simulink model "ABS_003"  (R2020b)
settings: Solver=VariableStepAuto  StartTime=0.0  StopTime=20  RelTol=1e-3
model workspace: external: MAT-File component_values.mat (data not in the file)
values from neighbouring files (symbols this model uses):
  g = 9.81    [component_values.mat]
  I = 5    [component_values.mat]
  m = 75    [component_values.mat]
  R = 1.25    [component_values.mat]
  Rr = 1.25    [component_values.mat]
  v0 = 44    [component_values.mat]
libraries: pid_lib x1
settings Model: Creator=Liu  LastModifiedBy=Quincy.liu
settings OptimizationCC: LifeSpan=inf
settings DebuggingCC: ArithmeticOperatorsInVariantConditions=warning
settings SFSimCC: CustomCodeUndefinedFunction=UseInterfaceOnly
settings CodeAppCC: StateflowObjectComments=on

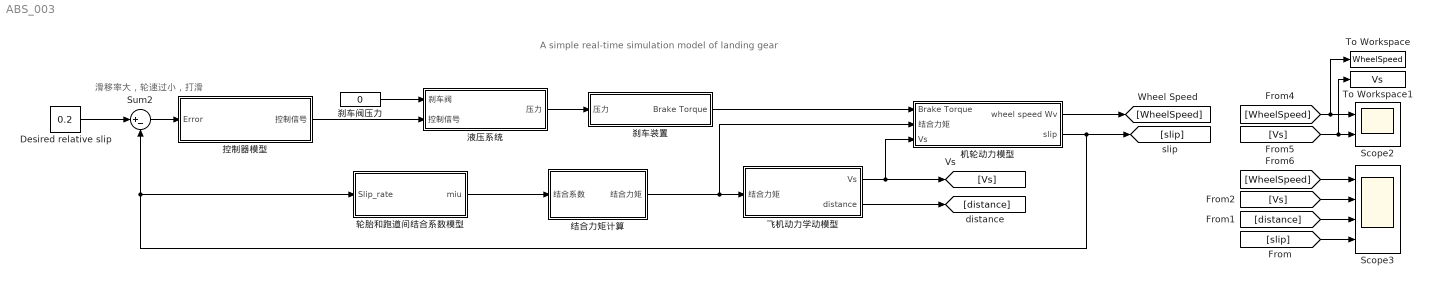
== system ABS_003 ==
  note: A simple real-time simulation model of landing gear
  note: 滑移率大，轮速过小，打滑
  Desired relative slip : Constant  Value=0.2
  Scope2 : Scope  NumInputPorts=2
  Scope3 : Scope  NumInputPorts=4
  Sum2 : Sum  Inputs=|+-  InputSameDT=on  SaturateOnIntegerOverflow=on  OutDataTypeStr=Inherit: Same as first input
  To Workspace : ToWorkspace  VariableName=WheelSpeed  SampleTime=-1
  To Workspace1 : ToWorkspace  VariableName=Vs  SaveFormat=Timeseries  SampleTime=-1
  刹车装置 : Subsystem
  刹车阀压力 : Constant  Value=0
  控制器模型 : Subsystem  Variant=on  VariantControlMode=label  LabelModeActiveChoice=Variant1
  "机轮动力模型 " : Subsystem
  液压系统 : Subsystem
  结合力矩计算 : Subsystem
  轮胎和跑道间结合系数模型 : Subsystem
  飞机动力学动模型 : Subsystem
  wires:
  Desired relative slip/1 -> Sum2/1
  结合力矩计算/1(结合力矩) -> 飞机动力学动模型/1(结合力矩), "机轮动力模型 "/2(结合力矩)
  轮胎和跑道间结合系数模型/1(miu) -> 结合力矩计算/1(结合系数)
  飞机动力学动模型/1(Vs) -> [Vs], "机轮动力模型 "/3(Vs)
  飞机动力学动模型/2(distance) -> [distance]
  Sum2/1 -> 控制器模型/1(Error)
  控制器模型/1(控制信号) -> 液压系统/2(控制信号)
  液压系统/1(压力) -> 刹车装置/1(压力)
  刹车装置/1(Brake Torque) -> "机轮动力模型 "/1(Brake Torque)
  "机轮动力模型 "/2(slip) -> [slip], 轮胎和跑道间结合系数模型/1(Slip_rate), Sum2/2
  [slip] -> Scope3/4
  [distance] -> Scope3/3
  [Vs] -> Scope3/2
  "机轮动力模型 "/1(wheel speed Wv) -> [WheelSpeed]
  [Vs] -> To Workspace1/1, Scope2/2
  [WheelSpeed] -> To Workspace/1, Scope2/1
  [WheelSpeed] -> Scope3/1
  刹车阀压力/1 -> 液压系统/1(刹车阀)

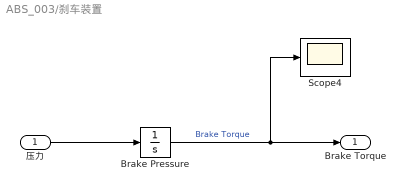
== system ABS_003/刹车装置 ==
  压力 : Inport
  Brake Pressure : Integrator  LimitOutput=on  UpperSaturationLimit=1000  LowerSaturationLimit=0
  Scope4 : Scope
  Brake Torque : Outport
  wires:
  Brake Pressure/1 -> Brake Torque/1, Scope4/1  "Brake Torque"
  压力/1 -> Brake Pressure/1

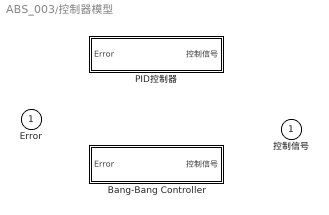
== system ABS_003/控制器模型 ==
  Error : Inport
  "Bang-Bang Controller " : Subsystem  VariantControl=Variant2
  PID控制器 : Subsystem  TreatAsAtomicUnit=on  VariantControl=Variant1
  控制信号 : Outport

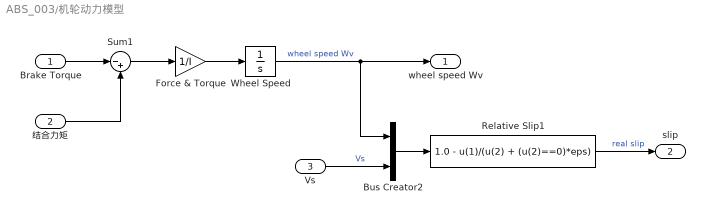
== system ABS_003/机轮动力模型  ==
  Brake Torque : Inport
  结合力矩 : Inport  Port=2
  Vs : Inport  Port=3
  Bus Creator2 : BusCreator  Inputs=2
  Force & Torque : Gain  Gain=1/I
  Relative Slip1 : Fcn  Expr=1.0 - u(1)/(u(2) + (u(2)==0)*eps)
  Sum1 : Sum  Inputs=|-+
  Wheel Speed : Integrator  InitialCondition=v0/R  LimitOutput=on  UpperSaturationLimit=1000  LowerSaturationLimit=0
  wheel speed Wv : Outport
  slip : Outport  Port=2
  wires:
  Force & Torque/1 -> Wheel Speed/1
  结合力矩/1 -> Sum1/2
  Sum1/1 -> Force & Torque/1
  Brake Torque/1 -> Sum1/1
  Vs/1 -> Bus Creator2/2  "Vs"
  Bus Creator2/1 -> Relative Slip1/1
  Relative Slip1/1 -> slip/1  "real slip"
  Wheel Speed/1 -> Bus Creator2/1, wheel speed Wv/1  "wheel speed Wv"

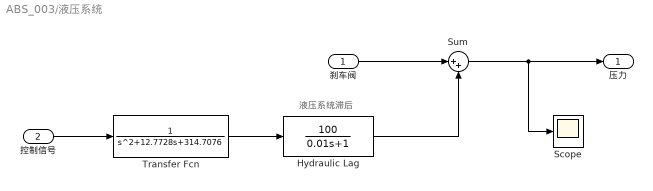
== system ABS_003/液压系统 ==
  note: 液压系统滞后
  刹车阀 : Inport
  控制信号 : Inport  Port=2
  Hydraulic Lag : TransferFcn  Numerator=[100]  Denominator=[0.01 1]
  Scope : Scope
  Sum : Sum  Inputs=|++
  Transfer Fcn : TransferFcn  Denominator=[1 12.7728 314.7076]
  压力 : Outport
  wires:
  控制信号/1 -> Transfer Fcn/1
  Transfer Fcn/1 -> Hydraulic Lag/1
  Hydraulic Lag/1 -> Sum/2
  刹车阀/1 -> Sum/1
  Sum/1 -> Scope/1, 压力/1

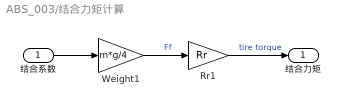
== system ABS_003/结合力矩计算 ==
  结合系数 : Inport
  Rr1 : Gain  Gain=Rr  SaturateOnIntegerOverflow=on  OutDataTypeStr=Inherit: Same as input  ParamDataTypeStr=Inherit: Same as input
  Weight1 : Gain  Gain=m*g/4  SaturateOnIntegerOverflow=on  OutDataTypeStr=Inherit: Same as input  ParamDataTypeStr=Inherit: Same as input
  结合力矩 : Outport
  wires:
  Weight1/1 -> Rr1/1  "Ff"
  Rr1/1 -> 结合力矩/1  "tire torque"
  结合系数/1 -> Weight1/1

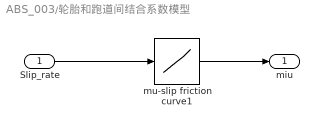
== system ABS_003/轮胎和跑道间结合系数模型 ==
  Slip_rate : Inport
  mu-slip friction curve1 : Lookup_n-D  NumberOfTableDimensions=1  BreakpointsForDimension1=|  Table=|  SaturateOnIntegerOverflow=on  InputSameDT=on
      BreakpointsForDimension1=|
      | [0
      | 0.05
      | 0.1
      | 0.15
      | 0.2
      | 0.25
      | 0.3
      | 0.35
      | 0.4
      | 0.45
      | 0.5
      | 0.55
      | 0.6
      | 0.65
      | 0.7
      | 0.75
      | 0.8
      | 0.85
      | 0.9
      | 0.95
      | 1
      | ]
      Table=|
      | [0
      | 0.4
      | 0.8
      | 0.97
      | 1
      | 0.98
      | 0.96
      | 0.94
      | 0.92
      | 0.9
      | 0.88
      | 0.855
      | 0.83
      | 0.81
      | 0.79
      | 0.77
      | 0.75
      | 0.73
      | 0.72
      | 0.71
      | 0.7
      | ]
  miu : Outport
  wires:
  mu-slip friction curve1/1 -> miu/1
  Slip_rate/1 -> mu-slip friction curve1/1

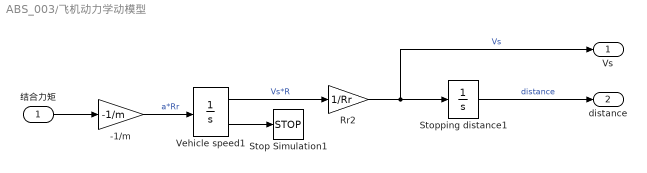
== system ABS_003/飞机动力学动模型 ==
  结合力矩 : Inport
  -1/m : Gain  Gain=-1/m  SaturateOnIntegerOverflow=on  OutDataTypeStr=Inherit: Same as input  ParamDataTypeStr=Inherit: Same as input
  Rr2 : Gain  Gain=1/Rr  SaturateOnIntegerOverflow=on  OutDataTypeStr=Inherit: Same as input  ParamDataTypeStr=Inherit: Same as input
  Stop Simulation1 : Stop
  Stopping distance1 : Integrator  UpperSaturationLimit=1000  LowerSaturationLimit=0
  Vehicle speed1 : Integrator  InitialCondition=v0  LimitOutput=on  UpperSaturationLimit=1000  LowerSaturationLimit=0  ShowSaturationPort=on
  Vs : Outport
  distance : Outport  Port=2
  wires:
  Rr2/1 -> Vs/1, Stopping distance1/1  "Vs"
  -1/m/1 -> Vehicle speed1/1  "a*Rr"
  Stopping distance1/1 -> distance/1  "distance"
  Vehicle speed1/2 -> Stop Simulation1/1
  Vehicle speed1/1 -> Rr2/1  "Vs*R"
  结合力矩/1 -> -1/m/1

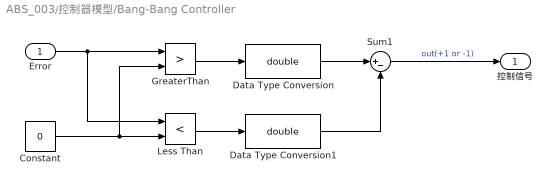
== system ABS_003/控制器模型/Bang-Bang Controller  ==
  Error : Inport
  Constant : Constant  Value=0
  Data Type Conversion : DataTypeConversion  OutDataTypeStr=double  RndMeth=Zero
  Data Type Conversion1 : DataTypeConversion  OutDataTypeStr=double  RndMeth=Zero
  GreaterThan : RelationalOperator  Operator=>  OutDataTypeStr=boolean  RndMeth=Nearest
  Less Than : RelationalOperator  Operator=<  OutDataTypeStr=boolean  RndMeth=Nearest
  Sum1 : Sum  Inputs=|+-
  控制信号 : Outport
  wires:
  Less Than/1 -> Data Type Conversion1/1
  Data Type Conversion1/1 -> Sum1/2
  Data Type Conversion/1 -> Sum1/1
  Constant/1 -> Less Than/2, GreaterThan/2
  Error/1 -> GreaterThan/1, Less Than/1
  Sum1/1 -> 控制信号/1  "out(+1 or -1)"
  GreaterThan/1 -> Data Type Conversion/1

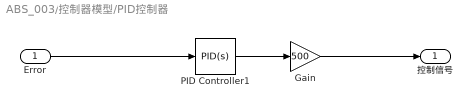
== system ABS_003/控制器模型/PID控制器 ==
  Error : Inport
  Gain : Gain  Gain=500
  PID Controller1 : pid_lib/PID Controller  Controller=PID  Form=Parallel  TimeDomain=Continuous-time  UseExternalTs=off  SampleTime=-1  IntegratorMethod=Forward Euler  FilterMethod=Forward Euler  ControllerParametersSource=internal  P=2  I=0  D=2  UseFilter=on  N=100  TunerSelectOption=Transfer Function Based (PID Tuner App)  InitialConditionSource=internal  InitialConditionForIntegrator=0  InitialConditionForFilter=0  DifferentiatorICPrevScaledInput=0  ExternalReset=none  TrackingMode=off  Kt=1  LimitOutput=off  SatLimitsSource=internal  UpperSaturationLimit=inf  LowerSaturationLimit=-inf  LinearizeAsGain=on  AntiWindupMode=none  Kb=1  POutMin=[]  POutMax=[]  IOutMin=[]  IOutMax=[]  DOutMin=[]  DOutMax=[]  NOutMin=[]  NOutMax=[]  SumOutMin=[]  SumOutMax=[]  SaturationOutMin=[]  SaturationOutMax=[]  PParamMin=[]  PParamMax=[]  IParamMin=[]  IParamMax=[]  DParamMin=[]  DParamMax=[]  NParamMin=[]  NParamMax=[]  KbParamMin=[]  KbParamMax=[]  KtParamMin=[]  KtParamMax=[]  KbOutMin=[]  KbOutMax=[]  KtOutMin=[]  KtOutMax=[]  IntegratorOutMin=[]  IntegratorOutMax=[]  FilterOutMin=[]  FilterOutMax=[]  SumI1OutMin=[]  SumI1OutMax=[]  SumI2OutMin=[]  SumI2OutMax=[]  SumI3OutMin=[]  SumI3OutMax=[]  SumI4OutMin=[]  SumI4OutMax=[]  SumDOutMin=[]  SumDOutMax=[]  DifferentiatorOutMin=[]  DifferentiatorOutMax=[]  FilterDiffOutCoefMin=[]  FilterDiffOutCoefMax=[]  ReciprocalOutMin=[]  ReciprocalOutMax=[]  SumDenOutMin=[]  SumDenOutMax=[]  SumNumOutMin=[]  SumNumOutMax=[]  DivideOutMin=[]  DivideOutMax=[]  UdiffTsProdOutMin=[]  UdiffTsProdOutMax=[]  NTsProdOutMin=[]  NTsProdOutMax=[]  UintegralTsProdOutMin=[]  UintegralTsProdOutMax=[]  UngainTsProdOutMin=[]  UngainTsProdOutMax=[]  IntegratorContinuousStateAttributes=''  IntegratorStateMustResolveToSignalObject=off  IntegratorRTWStateStorageClass=Auto  FilterContinuousStateAttributes=''  FilterStateMustResolveToSignalObject=off  FilterRTWStateStorageClass=Auto  ParallelPVariant=InternalParameters  IdealPVariant=Disabled  IVariant=InternalParameters  DVariant=InternalParameters  IntegratorVariant=Continuous  SatVariant=Disabled  AWVariant=Passthrough  PCopyVariant=Disabled  TRVariant=Disabled  FdbkBlocksVariant=Forward  IdealPFdbkVariant=Disabled  SatFdbkVariant=Disabled  DerivativeFilterVariant=ContFilter  NVariant=InternalParameters  NCopyVariant=Disabled  FilterICVariant=InternalICsFilter  IntegratorICVariant=InternalICs  ExternalResetVariant=Disabled  TRSumVariant=Passthrough  SumFdbkVariant=Disabled  SumVariant=Sum_PID  TsampFilterVariant=InternalTs  TsampNgainVariant=Passthrough  TsampIntegralVariant=Passthrough  ExternalSaturationOutDataTypeStr=Inherit: Same as second input
  控制信号 : Outport
  wires:
  PID Controller1/1 -> Gain/1
  Error/1 -> PID Controller1/1
  Gain/1 -> 控制信号/1
